simulink subsystem "Orbit_controller"  (R2020a)
settings: Solver=VariableStepAuto  StartTime=0.0  StopTime=10.0  RelTol=1e-3
settings Model: Creator=decla  LastModifiedBy=decla

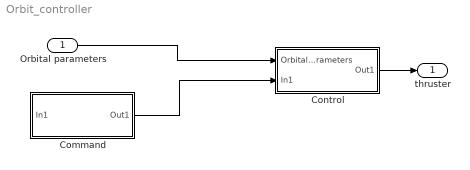
== system Orbit_controller ==
  Orbital parameters : Inport
  Command : Subsystem
  Control : Subsystem
  thruster : Outport
  wires:
  Control/1(Out1) -> thruster/1
  Orbital parameters/1 -> Control/1(Orbital parameters)
  Command/1(Out1) -> Control/2(In1)

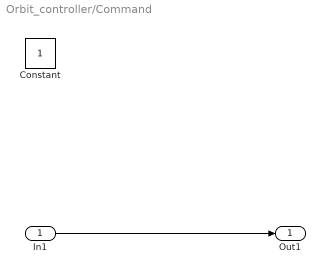
== system Orbit_controller/Command ==
  In1 : Inport
  Constant : Constant
  Out1 : Outport
  wires:
  In1/1 -> Out1/1

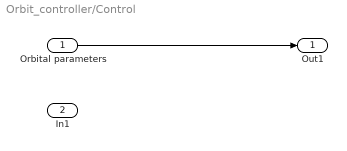
== system Orbit_controller/Control ==
  Orbital parameters : Inport
  In1 : Inport  Port=2
  Out1 : Outport
  wires:
  Orbital parameters/1 -> Out1/1
